simulink model "simulink_display"  (R2013a)
settings: Solver=ode45  StartTime=0.0  StopTime=10.0  RelTol=1e-3
settings Model: Creator=alper pc  LastModifiedBy=alper pc

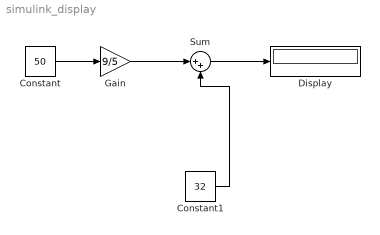
== system simulink_display ==
  Constant : Constant  Value=50
  Constant1 : Constant  Value=32
  Display : Display
  Gain : Gain  Gain=9/5
  Sum : Sum  Inputs=|++
  wires:
  Constant1/1 -> Sum/2
  Constant/1 -> Gain/1
  Gain/1 -> Sum/1
  Sum/1 -> Display/1
